simulink model "dcBusPITuningRL"  (R2025b)
settings: Solver=ode4  StartTime=0.0  StopTime=1.0  FixedStep=0.001  RelTol=1e-3
libraries: simulink x1, rllib x1
settings Model: Creator=Santhosh  LastModifiedBy=Santhosh

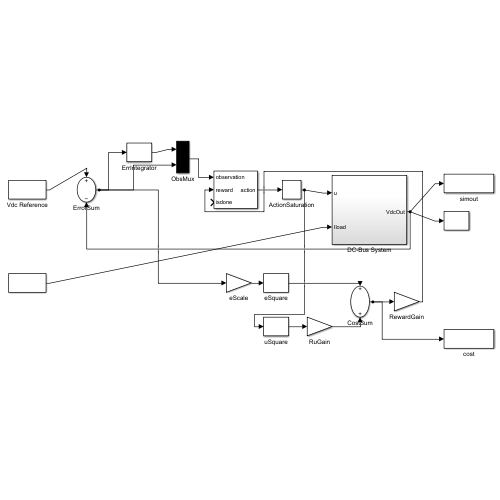
[thumbnail: Simulink's stored preview of the top-level diagram]
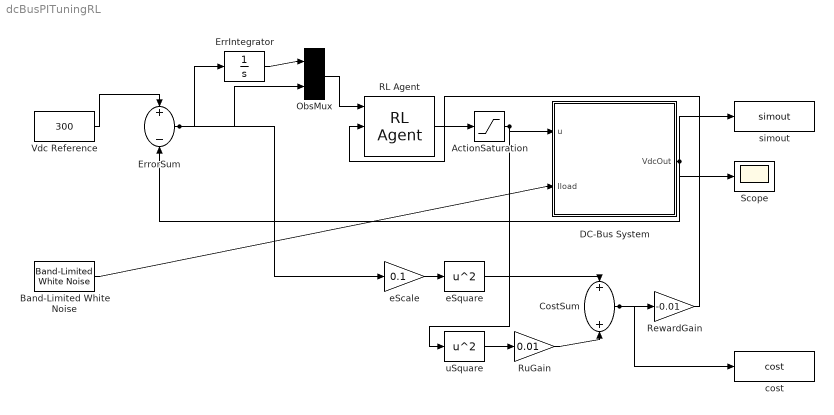
== system dcBusPITuningRL ==
  ActionSaturation : Saturate  UpperLimit=10.0503  LowerLimit=-9.3339
  Band-Limited White Noise : simulink/Sources/Band-Limited White Noise  Cov=5  Ts=0.001  seed=23341
  CostSum : Sum
  DC-Bus System : Subsystem
  ErrIntegrator : Integrator
  ErrorSum : Sum  Inputs=+-
  ObsMux : Mux  Inputs=2
  RL Agent : rllib/RL Agent  Agent=agentObj  ExternalActionAsInput=off  ProvideLastAction=off  ProvideCumRwd=off  TreatAsDirectFeedthrough=on  UseStrictObservationDataTypes=off
  RewardGain : Gain  Gain=-0.01
  RuGain : Gain  Gain=0.01
  Scope : Scope
  Vdc Reference : Constant  Value=300
  cost : ToWorkspace  VariableName=cost  SaveFormat=Timeseries  SampleTime=-1
  eScale : Gain  Gain=0.1
  eSquare : Math  Operator=square
  simout : ToWorkspace  VariableName=simout  SaveFormat=Timeseries  SampleTime=-1
  uSquare : Math  Operator=square
  wires:
  Vdc Reference/1 -> ErrorSum/1
  DC-Bus System/1(VdcOut) -> ErrorSum/2, simout/1, Scope/1
  ErrorSum/1 -> ErrIntegrator/1, ObsMux/2, eScale/1
  ErrIntegrator/1 -> ObsMux/1
  ObsMux/1 -> RL Agent/1
  RewardGain/1 -> RL Agent/2
  RL Agent/1 -> ActionSaturation/1
  ActionSaturation/1 -> DC-Bus System/1(u), uSquare/1
  Band-Limited White Noise/1 -> DC-Bus System/2(Iload)
  eScale/1 -> eSquare/1
  uSquare/1 -> RuGain/1
  eSquare/1 -> CostSum/1
  RuGain/1 -> CostSum/2
  CostSum/1 -> RewardGain/1, cost/1

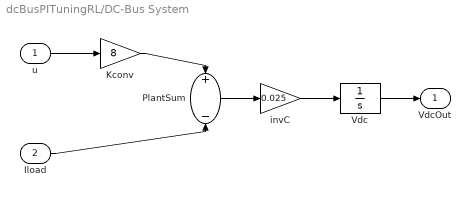
== system dcBusPITuningRL/DC-Bus System ==
  u : Inport
  Iload : Inport  Port=2
  Kconv : Gain  Gain=8
  PlantSum : Sum  Inputs=+-
  Vdc : Integrator  InitialCondition=297.9049
  invC : Gain  Gain=0.025
  VdcOut : Outport
  wires:
  u/1 -> Kconv/1
  Kconv/1 -> PlantSum/1
  Iload/1 -> PlantSum/2
  PlantSum/1 -> invC/1
  invC/1 -> Vdc/1
  Vdc/1 -> VdcOut/1
